simulink library "VIS_LIB"  (Simulink 8.6)
settings: Solver=ode45  StartTime=0.0  StopTime=10.0  RelTol=1e-3
undefined symbols (not defined in the file): AC, SIXOSEM_F_WD_AC_MASTER
libraries: cdsFilt x376, cdsEpicsOut x253, cdsEpicsIn x179, cdsTP x123, VIS_LIB x95, cdsMuxMatrix x91, cdsEpicsStringIn x75, cdsFiltCtrl x72, cdsFunctionCall x70, cdsRms x59, KAGRA_UTIL x25, STATE_BIO_MASTER x5
(part 5 of 38)

== system VIS_LIB/OLDAMP ==
  note: 1 (one) if GOOD
      | 0 (zero) if BAD
  PITCH_In : Inport
  YAW_In : Inport  Port=2
  Ground{1..2,4..5} (4 alike) : Ground
  Operator4 : RelationalOperator  Operator===  OutDataTypeStr=boolean
  Operator5 : RelationalOperator  Operator===  OutDataTypeStr=boolean
  P : cdsFiltCtrl/IIR FM with control  Tag=cdsFiltCtrl  Description=|
      | cdsFiltCntrl is the standard IIR filter module (exactly the same as cdsFilt) but with added control data output 'Ctrl'. Filter module digital signal output appears on the first output, which is called 'Val'. 'Ctrl' output has a bit pattern encoding the state of filter's on/off switches (FM1 through FM10). The bit values are:
      |                                                                                                                                                                                                                                                                                                                                       
      | module 	hex	dec                                                                                                                                                                                                                                                                                                                       
      | -----------------------                                                                                                                                                                                                                                                                                                               
      | FM1	0x20                    32                                                                                                                                                                                                                                                                                                        
      | FM2	0x80                     128                                                                                                                                                                                                                                                                                                      
      | FM3	0x200                   512                                                                                                                                                                                                                                                                                                       
      | FM4	0x800                   2048                                                                                                                                                                                                                                                                                                      
      | FM5	0x2000                 8192                                                                                                                                                                                                                                                                                                       
      | FM6	0x8000                 32768                                                                                                                                                                                                                                                                                                      
      | FM7	0x20000                131072                                                                                                                                                                                                                                                                                                     
      | FM8	0x80000                 524288                                                                                                                                                                                                                                                                                                    
      | FM9	0x200000               2097152                                                                                                                                                                                                                                                                                                    
      | FM10	0x800000               8388608                                                                                                                                                                                                                                                                                                   
      |                                                                                                                                                                                                                                                                                                                                       
      | This bit data can be used to drive some other switches or it can be output using a binary I/O module.
      settings: AttributesFormatString=%<Tag>
  P_STATE_GOOD : cdsEpicsIn/Subsystem  Tag=cdsEpicsIn  Description=|
      | Purpose:                                                                              
      | Create an EPICS input channel connection to the FE realtime controls.                 
      |                                                                                       
      | Operation:                                                                            
      | Outputs value from an EPICS ai record. Value is floating point with a precision of 3..
      |                                                                                       
      | Usage:                                                                                
      | Name the part with the desired EPICS channel name.
      settings: AttributesFormatString=%<Tag>
  P_STATE_NOW : cdsEpicsOut/Subsystem  Tag=cdsEpicsOutput  Description=|
      | Purpose:                                          
      | Output a FE signal to an EPICS channel.           
      |                                                   
      | Operation:                                        
      | Takes input value and passes it to EPICS record.  
      |                                                   
      | Usage:                                            
      | Name the part with the desired EPICS rrecord name.
      settings: AttributesFormatString=%<Tag>
  P_STATE_OK : cdsEpicsOut/Subsystem  Tag=cdsEpicsOutput  Description=|
      | Purpose:                                          
      | Output a FE signal to an EPICS channel.           
      |                                                   
      | Operation:                                        
      | Takes input value and passes it to EPICS record.  
      |                                                   
      | Usage:                                            
      | Name the part with the desired EPICS rrecord name.
      settings: AttributesFormatString=%<Tag>
  Product : Product  RndMeth=Zero
  STATE_OK : cdsEpicsOut/Subsystem  Tag=cdsEpicsOutput  Description=|
      | Purpose:                                          
      | Output a FE signal to an EPICS channel.           
      |                                                   
      | Operation:                                        
      | Takes input value and passes it to EPICS record.  
      |                                                   
      | Usage:                                            
      | Name the part with the desired EPICS rrecord name.
      settings: AttributesFormatString=%<Tag>
  Y : cdsFiltCtrl/IIR FM with control  Tag=cdsFiltCtrl  Description=|
      | cdsFiltCntrl is the standard IIR filter module (exactly the same as cdsFilt) but with added control data output 'Ctrl'. Filter module digital signal output appears on the first output, which is called 'Val'. 'Ctrl' output has a bit pattern encoding the state of filter's on/off switches (FM1 through FM10). The bit values are:
      |                                                                                                                                                                                                                                                                                                                                       
      | module 	hex	dec                                                                                                                                                                                                                                                                                                                       
      | -----------------------                                                                                                                                                                                                                                                                                                               
      | FM1	0x20                    32                                                                                                                                                                                                                                                                                                        
      | FM2	0x80                     128                                                                                                                                                                                                                                                                                                      
      | FM3	0x200                   512                                                                                                                                                                                                                                                                                                       
      | FM4	0x800                   2048                                                                                                                                                                                                                                                                                                      
      | FM5	0x2000                 8192                                                                                                                                                                                                                                                                                                       
      | FM6	0x8000                 32768                                                                                                                                                                                                                                                                                                      
      | FM7	0x20000                131072                                                                                                                                                                                                                                                                                                     
      | FM8	0x80000                 524288                                                                                                                                                                                                                                                                                                    
      | FM9	0x200000               2097152                                                                                                                                                                                                                                                                                                    
      | FM10	0x800000               8388608                                                                                                                                                                                                                                                                                                   
      |                                                                                                                                                                                                                                                                                                                                       
      | This bit data can be used to drive some other switches or it can be output using a binary I/O module.
      settings: AttributesFormatString=%<Tag>
  Y_STATE_GOOD : cdsEpicsIn/Subsystem  Tag=cdsEpicsIn  Description=|
      | Purpose:                                                                              
      | Create an EPICS input channel connection to the FE realtime controls.                 
      |                                                                                       
      | Operation:                                                                            
      | Outputs value from an EPICS ai record. Value is floating point with a precision of 3..
      |                                                                                       
      | Usage:                                                                                
      | Name the part with the desired EPICS channel name.
      settings: AttributesFormatString=%<Tag>
  Y_STATE_NOW : cdsEpicsOut/Subsystem  Tag=cdsEpicsOutput  Description=|
      | Purpose:                                          
      | Output a FE signal to an EPICS channel.           
      |                                                   
      | Operation:                                        
      | Takes input value and passes it to EPICS record.  
      |                                                   
      | Usage:                                            
      | Name the part with the desired EPICS rrecord name.
      settings: AttributesFormatString=%<Tag>
  Y_STATE_OK : cdsEpicsOut/Subsystem  Tag=cdsEpicsOutput  Description=|
      | Purpose:                                          
      | Output a FE signal to an EPICS channel.           
      |                                                   
      | Operation:                                        
      | Takes input value and passes it to EPICS record.  
      |                                                   
      | Usage:                                            
      | Name the part with the desired EPICS rrecord name.
      settings: AttributesFormatString=%<Tag>
  PITCH_Out : Outport
  YAW_Out : Outport  Port=2
  OLDAMP_STATE_Out : Outport  Port=3
  wires:
  Ground2/1 -> Y/3
  Ground1/1 -> P/3
  P/1 -> PITCH_Out/1
  Ground4/1 -> P/2
  PITCH_In/1 -> P/1
  P_STATE_GOOD/1 -> Operator4/1
  P/2 -> P_STATE_NOW/1
  Ground5/1 -> Y/2
  YAW_In/1 -> Y/1
  Y_STATE_GOOD/1 -> Operator5/1
  Y/2 -> Y_STATE_NOW/1
  Y/1 -> YAW_Out/1
  Operator4/1 -> P_STATE_OK/1
  Operator5/1 -> Y_STATE_OK/1
  Product/1 -> STATE_OK/1
  P_STATE_NOW/1 -> Operator4/2
  Y_STATE_NOW/1 -> Operator5/2
  STATE_OK/1 -> OLDAMP_STATE_Out/1
  P_STATE_OK/1 -> Product/1
  Y_STATE_OK/1 -> Product/2

== system VIS_LIB/OLDCCTRL ==
  note: 1 (one) if GOOD
      | 0 (zero) if BAD
  PITCH_In : Inport
  YAW_In : Inport  Port=2
  Ground{1..2,4..5} (4 alike) : Ground
  Operator4 : RelationalOperator  Operator===  OutDataTypeStr=boolean
  Operator5 : RelationalOperator  Operator===  OutDataTypeStr=boolean
  P : cdsFiltCtrl/IIR FM with control  Tag=cdsFiltCtrl  Description=|
      | cdsFiltCntrl is the standard IIR filter module (exactly the same as cdsFilt) but with added control data output 'Ctrl'. Filter module digital signal output appears on the first output, which is called 'Val'. 'Ctrl' output has a bit pattern encoding the state of filter's on/off switches (FM1 through FM10). The bit values are:
      |                                                                                                                                                                                                                                                                                                                                       
      | module 	hex	dec                                                                                                                                                                                                                                                                                                                       
      | -----------------------                                                                                                                                                                                                                                                                                                               
      | FM1	0x20                    32                                                                                                                                                                                                                                                                                                        
      | FM2	0x80                     128                                                                                                                                                                                                                                                                                                      
      | FM3	0x200                   512                                                                                                                                                                                                                                                                                                       
      | FM4	0x800                   2048                                                                                                                                                                                                                                                                                                      
      | FM5	0x2000                 8192                                                                                                                                                                                                                                                                                                       
      | FM6	0x8000                 32768                                                                                                                                                                                                                                                                                                      
      | FM7	0x20000                131072                                                                                                                                                                                                                                                                                                     
      | FM8	0x80000                 524288                                                                                                                                                                                                                                                                                                    
      | FM9	0x200000               2097152                                                                                                                                                                                                                                                                                                    
      | FM10	0x800000               8388608                                                                                                                                                                                                                                                                                                   
      |                                                                                                                                                                                                                                                                                                                                       
      | This bit data can be used to drive some other switches or it can be output using a binary I/O module.
      settings: AttributesFormatString=%<Tag>
  P_STATE_GOOD : cdsEpicsIn/Subsystem  Tag=cdsEpicsIn  Description=|
      | Purpose:                                                                              
      | Create an EPICS input channel connection to the FE realtime controls.                 
      |                                                                                       
      | Operation:                                                                            
      | Outputs value from an EPICS ai record. Value is floating point with a precision of 3..
      |                                                                                       
      | Usage:                                                                                
      | Name the part with the desired EPICS channel name.
      settings: AttributesFormatString=%<Tag>
  P_STATE_NOW : cdsEpicsOut/Subsystem  Tag=cdsEpicsOutput  Description=|
      | Purpose:                                          
      | Output a FE signal to an EPICS channel.           
      |                                                   
      | Operation:                                        
      | Takes input value and passes it to EPICS record.  
      |                                                   
      | Usage:                                            
      | Name the part with the desired EPICS rrecord name.
      settings: AttributesFormatString=%<Tag>
  P_STATE_OK : cdsEpicsOut/Subsystem  Tag=cdsEpicsOutput  Description=|
      | Purpose:                                          
      | Output a FE signal to an EPICS channel.           
      |                                                   
      | Operation:                                        
      | Takes input value and passes it to EPICS record.  
      |                                                   
      | Usage:                                            
      | Name the part with the desired EPICS rrecord name.
      settings: AttributesFormatString=%<Tag>
  Product : Product  RndMeth=Zero
  STATE_OK : cdsEpicsOut/Subsystem  Tag=cdsEpicsOutput  Description=|
      | Purpose:                                          
      | Output a FE signal to an EPICS channel.           
      |                                                   
      | Operation:                                        
      | Takes input value and passes it to EPICS record.  
      |                                                   
      | Usage:                                            
      | Name the part with the desired EPICS rrecord name.
      settings: AttributesFormatString=%<Tag>
  Y : cdsFiltCtrl/IIR FM with control  Tag=cdsFiltCtrl  Description=|
      | cdsFiltCntrl is the standard IIR filter module (exactly the same as cdsFilt) but with added control data output 'Ctrl'. Filter module digital signal output appears on the first output, which is called 'Val'. 'Ctrl' output has a bit pattern encoding the state of filter's on/off switches (FM1 through FM10). The bit values are:
      |                                                                                                                                                                                                                                                                                                                                       
      | module 	hex	dec                                                                                                                                                                                                                                                                                                                       
      | -----------------------                                                                                                                                                                                                                                                                                                               
      | FM1	0x20                    32                                                                                                                                                                                                                                                                                                        
      | FM2	0x80                     128                                                                                                                                                                                                                                                                                                      
      | FM3	0x200                   512                                                                                                                                                                                                                                                                                                       
      | FM4	0x800                   2048                                                                                                                                                                                                                                                                                                      
      | FM5	0x2000                 8192                                                                                                                                                                                                                                                                                                       
      | FM6	0x8000                 32768                                                                                                                                                                                                                                                                                                      
      | FM7	0x20000                131072                                                                                                                                                                                                                                                                                                     
      | FM8	0x80000                 524288                                                                                                                                                                                                                                                                                                    
      | FM9	0x200000               2097152                                                                                                                                                                                                                                                                                                    
      | FM10	0x800000               8388608                                                                                                                                                                                                                                                                                                   
      |                                                                                                                                                                                                                                                                                                                                       
      | This bit data can be used to drive some other switches or it can be output using a binary I/O module.
      settings: AttributesFormatString=%<Tag>
  Y_STATE_GOOD : cdsEpicsIn/Subsystem  Tag=cdsEpicsIn  Description=|
      | Purpose:                                                                              
      | Create an EPICS input channel connection to the FE realtime controls.                 
      |                                                                                       
      | Operation:                                                                            
      | Outputs value from an EPICS ai record. Value is floating point with a precision of 3..
      |                                                                                       
      | Usage:                                                                                
      | Name the part with the desired EPICS channel name.
      settings: AttributesFormatString=%<Tag>
  Y_STATE_NOW : cdsEpicsOut/Subsystem  Tag=cdsEpicsOutput  Description=|
      | Purpose:                                          
      | Output a FE signal to an EPICS channel.           
      |                                                   
      | Operation:                                        
      | Takes input value and passes it to EPICS record.  
      |                                                   
      | Usage:                                            
      | Name the part with the desired EPICS rrecord name.
      settings: AttributesFormatString=%<Tag>
  Y_STATE_OK : cdsEpicsOut/Subsystem  Tag=cdsEpicsOutput  Description=|
      | Purpose:                                          
      | Output a FE signal to an EPICS channel.           
      |                                                   
      | Operation:                                        
      | Takes input value and passes it to EPICS record.  
      |                                                   
      | Usage:                                            
      | Name the part with the desired EPICS rrecord name.
      settings: AttributesFormatString=%<Tag>
  PITCH_Out : Outport
  YAW_Out : Outport  Port=2
  OLDCCTRL_STATE_Out : Outport  Port=3
  wires:
  Ground2/1 -> Y/3
  Ground1/1 -> P/3
  P/1 -> PITCH_Out/1
  Ground4/1 -> P/2
  PITCH_In/1 -> P/1
  P_STATE_GOOD/1 -> Operator4/1
  P/2 -> P_STATE_NOW/1
  Ground5/1 -> Y/2
  YAW_In/1 -> Y/1
  Y_STATE_GOOD/1 -> Operator5/1
  Y/2 -> Y_STATE_NOW/1
  Y/1 -> YAW_Out/1
  Operator4/1 -> P_STATE_OK/1
  Operator5/1 -> Y_STATE_OK/1
  Product/1 -> STATE_OK/1
  P_STATE_NOW/1 -> Operator4/2
  Y_STATE_NOW/1 -> Operator5/2
  STATE_OK/1 -> OLDCCTRL_STATE_Out/1
  P_STATE_OK/1 -> Product/1
  Y_STATE_OK/1 -> Product/2

== system VIS_LIB/OPLEV_BLRMS_DOF ==
  In1 : Inport
  100M_300M : cdsEpicsOut/Subsystem  Tag=cdsEpicsOutput  Description=|
      | Purpose:                                          
      | Output a FE signal to an EPICS channel.           
      |                                                   
      | Operation:                                        
      | Takes input value and passes it to EPICS record.  
      |                                                   
      | Usage:                                            
      | Name the part with the desired EPICS rrecord name.
      settings: AttributesFormatString=%<Tag>
  10_30 : cdsEpicsOut/Subsystem  Tag=cdsEpicsOutput  Description=|
      | Purpose:                                          
      | Output a FE signal to an EPICS channel.           
      |                                                   
      | Operation:                                        
      | Takes input value and passes it to EPICS record.  
      |                                                   
      | Usage:                                            
      | Name the part with the desired EPICS rrecord name.
      settings: AttributesFormatString=%<Tag>
  1_3 : cdsEpicsOut/Subsystem  Tag=cdsEpicsOutput  Description=|
      | Purpose:                                          
      | Output a FE signal to an EPICS channel.           
      |                                                   
      | Operation:                                        
      | Takes input value and passes it to EPICS record.  
      |                                                   
      | Usage:                                            
      | Name the part with the desired EPICS rrecord name.
      settings: AttributesFormatString=%<Tag>
  300M_1 : cdsEpicsOut/Subsystem  Tag=cdsEpicsOutput  Description=|
      | Purpose:                                          
      | Output a FE signal to an EPICS channel.           
      |                                                   
      | Operation:                                        
      | Takes input value and passes it to EPICS record.  
      |                                                   
      | Usage:                                            
      | Name the part with the desired EPICS rrecord name.
      settings: AttributesFormatString=%<Tag>
  30M : cdsEpicsOut/Subsystem  Tag=cdsEpicsOutput  Description=|
      | Purpose:                                          
      | Output a FE signal to an EPICS channel.           
      |                                                   
      | Operation:                                        
      | Takes input value and passes it to EPICS record.  
      |                                                   
      | Usage:                                            
      | Name the part with the desired EPICS rrecord name.
      settings: AttributesFormatString=%<Tag>
  30M_100M : cdsEpicsOut/Subsystem  Tag=cdsEpicsOutput  Description=|
      | Purpose:                                          
      | Output a FE signal to an EPICS channel.           
      |                                                   
      | Operation:                                        
      | Takes input value and passes it to EPICS record.  
      |                                                   
      | Usage:                                            
      | Name the part with the desired EPICS rrecord name.
      settings: AttributesFormatString=%<Tag>
  30_100 : cdsEpicsOut/Subsystem  Tag=cdsEpicsOutput  Description=|
      | Purpose:                                          
      | Output a FE signal to an EPICS channel.           
      |                                                   
      | Operation:                                        
      | Takes input value and passes it to EPICS record.  
      |                                                   
      | Usage:                                            
      | Name the part with the desired EPICS rrecord name.
      settings: AttributesFormatString=%<Tag>
  3_10 : cdsEpicsOut/Subsystem  Tag=cdsEpicsOutput  Description=|
      | Purpose:                                          
      | Output a FE signal to an EPICS channel.           
      |                                                   
      | Operation:                                        
      | Takes input value and passes it to EPICS record.  
      |                                                   
      | Usage:                                            
      | Name the part with the desired EPICS rrecord name.
      settings: AttributesFormatString=%<Tag>
  BLRMS : cdsFunctionCall/Subsystem  Tag=cdsFunctionCall  Description=inline BLRMS /opt/rtcds/userapps/release/cds/common/src/BLRMSFILTER.c
      settings: AttributesFormatString=%<Tag>\n%<Description>
  Constant2 : Constant  Value=2
  Demux : Demux  Outputs=8
  Mux : Mux  Inputs=2
  Terminator{1..8} (8 alike) : Terminator
  wires:
  BLRMS/1 -> Demux/1
  Mux/1 -> BLRMS/1
  In1/1 -> Mux/1
  Demux/1 -> 30M/1
  Demux/2 -> 30M_100M/1
  Demux/3 -> 100M_300M/1
  Demux/4 -> 300M_1/1
  Demux/5 -> 1_3/1
  Demux/6 -> 3_10/1
  Demux/7 -> 10_30/1
  Demux/8 -> 30_100/1
  30M/1 -> Terminator8/1
  30M_100M/1 -> Terminator1/1
  100M_300M/1 -> Terminator2/1
  300M_1/1 -> Terminator3/1
  1_3/1 -> Terminator4/1
  3_10/1 -> Terminator5/1
  10_30/1 -> Terminator6/1
  30_100/1 -> Terminator7/1
  Constant2/1 -> Mux/2

== system VIS_LIB/PAY_OLSERVO ==
  OL_MNP_In : Inport
  OL_MNY_In : Inport  Port=2
  OL_TML_In : Inport  Port=3
  OL_TMP_In : Inport  Port=4
  OL_TMY_In : Inport  Port=5
  ADD : Subsystem
  DAMP : Subsystem
  Demux1 : Demux  Outputs=24
  Demux2 : Demux  Outputs=10
  Mux1 : Mux  Inputs=24
  Mux2 : Mux  Inputs=5
  OL2PK : cdsMuxMatrix/Subsystem  Tag=cdsMuxMatrix  Description=Any size matrix. Inputs and outputs must be connected using Mux and Demux parts.
      settings: AttributesFormatString=%<Tag>
  PK2EUL : cdsMuxMatrix/Subsystem  Tag=cdsMuxMatrix  Description=Any size matrix. Inputs and outputs must be connected using Mux and Demux parts.
      settings: AttributesFormatString=%<Tag>
  PKOUT : Subsystem
  TEST : Subsystem
  BFY_Out : Outport
  MNL_Out : Outport  Port=2
  MNP_Out : Outport  Port=3
  MNY_Out : Outport  Port=4
  IML_Out : Outport  Port=5
  IMP_Out : Outport  Port=6
  IMY_Out : Outport  Port=7
  TML_Out : Outport  Port=8
  TMP_Out : Outport  Port=9
  TMY_Out : Outport  Port=10
  wires:
  OL_TMP_In/1 -> Mux2/4
  OL_TMY_In/1 -> Mux2/5
  OL_MNP_In/1 -> Mux2/1
  OL_MNY_In/1 -> Mux2/2
  OL_TML_In/1 -> Mux2/3
  Mux2/1 -> OL2PK/1
  OL2PK/1 -> Demux1/1
  Demux1/3 -> DAMP/3(P03_In)
  Demux1/6 -> DAMP/6(P06_In)
  Demux1/4 -> DAMP/4(P04_In)
  Demux1/1 -> DAMP/1(P01_In)
  Demux1/2 -> DAMP/2(P02_In)
  Demux1/7 -> DAMP/7(P07_In)
  Demux1/8 -> DAMP/8(P08_In)
  Demux1/9 -> DAMP/9(P09_In)
  Demux1/10 -> DAMP/10(P10_In)
  Demux1/11 -> DAMP/11(P11_In)
  Demux1/12 -> DAMP/12(P12_In1)
  Demux1/5 -> DAMP/5(P05_In)
  TEST/12(P12_Out) -> ADD/12(TEST_P12_In)
  TEST/6(P06_Out) -> ADD/6(TEST_P06_In)
  TEST/7(P07_Out) -> ADD/7(TEST_P07_In)
  TEST/8(P08_Out) -> ADD/8(TEST_P08_In)
  TEST/9(P09_Out) -> ADD/9(TEST_P09_In)
  TEST/10(P10_Out) -> ADD/10(TEST_P10_In)
  TEST/11(P11_Out) -> ADD/11(TEST_P11_In)
  TEST/1(P01_Out) -> ADD/1(TEST_P01_In)
  TEST/2(P02_Out) -> ADD/2(TEST_P02_In)
  TEST/3(P03_Out) -> ADD/3(TEST_P03_In)
  TEST/4(P04_Out) -> ADD/4(TEST_P04_In)
  TEST/5(P05_Out) -> ADD/5(TEST_P05_In)
  DAMP/11(P11_Out) -> ADD/35(DAMP_P11_In)
  DAMP/4(P04_Out) -> ADD/28(DAMP_P04_In)
  DAMP/5(P05_Out) -> ADD/29(DAMP_P05_In)
  DAMP/6(P06_Out) -> ADD/30(DAMP_P06_In)
  DAMP/12(P12_Out) -> ADD/36(DAMP_P12_In)
  DAMP/8(P08_Out) -> ADD/32(DAMP_P08_In)
  DAMP/10(P10_Out) -> ADD/34(DAMP_P10_In)
  DAMP/7(P07_Out) -> ADD/31(DAMP_P07_In)
  DAMP/9(P09_Out) -> ADD/33(DAMP_P09_In)
  DAMP/1(P01_Out) -> ADD/25(DAMP_P01_In)
  DAMP/2(P02_Out) -> ADD/26(DAMP_P02_In)
  DAMP/3(P03_Out) -> ADD/27(DAMP_P03_In)
  Mux1/1 -> PK2EUL/1
  PK2EUL/1 -> Demux2/1
  Demux2/3 -> MNP_Out/1
  Demux2/1 -> BFY_Out/1
  Demux2/2 -> MNL_Out/1
  Demux2/10 -> TMY_Out/1
  Demux2/8 -> TML_Out/1
  Demux2/4 -> MNY_Out/1
  Demux2/9 -> TMP_Out/1
  Demux2/7 -> IMY_Out/1
  Demux2/5 -> IML_Out/1
  Demux2/6 -> IMP_Out/1
  Demux1/13 -> DAMP/13(P13_In)
  Demux1/14 -> DAMP/14(P14_In)
  Demux1/15 -> DAMP/15(P15_In)
  Demux1/16 -> DAMP/16(P16_In)
  Demux1/17 -> DAMP/17(P17_In)
  Demux1/18 -> DAMP/18(P18_In)
  Demux1/19 -> DAMP/19(P19_In)
  Demux1/20 -> DAMP/20(P20_In)
  Demux1/21 -> DAMP/21(P21_In)
  Demux1/22 -> DAMP/22(P22_In)
  Demux1/23 -> DAMP/23(P23_In)
  Demux1/24 -> DAMP/24(P24_In)
  TEST/13(P13_Out) -> ADD/13(TEST_P13_In)
  TEST/14(P14_Out) -> ADD/14(TEST_P14_In)
  TEST/15(P15_Out) -> ADD/15(TEST_P15_In)
  TEST/16(P16_Out) -> ADD/16(TEST_P16_In)
  TEST/17(P17_Out) -> ADD/17(TEST_P17_In)
  TEST/18(P18_Out) -> ADD/18(TEST_P18_In)
  TEST/19(P19_Out) -> ADD/19(TEST_P19_In)
  TEST/20(P20_Out) -> ADD/20(TEST_P20_In)
  TEST/21(P21_Out) -> ADD/21(TEST_P21_In)
  TEST/22(P22_Out) -> ADD/22(TEST_P22_In)
  TEST/23(P23_Out) -> ADD/23(TEST_P23_In)
  TEST/24(P24_Out) -> ADD/24(TEST_P24_In)
  DAMP/13(P13_Out) -> ADD/37(DAMP_P13_In)
  DAMP/14(P14_Out) -> ADD/38(DAMP_P14_In)
  DAMP/15(P15_Out) -> ADD/39(DAMP_P15_In)
  DAMP/16(P16_Out) -> ADD/40(DAMP_P16_In)
  DAMP/17(P17_Out) -> ADD/41(DAMP_P17_In)
  DAMP/18(P18_Out) -> ADD/42(DAMP_P18_In)
  DAMP/19(P19_Out) -> ADD/43(DAMP_P19_In)
  DAMP/20(P20_Out) -> ADD/44(DAMP_P20_In)
  DAMP/21(P21_Out) -> ADD/45(DAMP_P21_In)
  DAMP/22(P22_Out) -> ADD/46(DAMP_P22_In)
  DAMP/23(P23_Out) -> ADD/47(DAMP_P23_In)
  DAMP/24(P24_Out) -> ADD/48(DAMP_P24_In)
  ADD/16(P16_Out) -> PKOUT/16(P16_In), Mux1/16
  ADD/14(P14_Out) -> PKOUT/14(P14_In), Mux1/14
  ADD/19(P19_Out) -> PKOUT/19(P19_In), Mux1/19
  ADD/20(P20_Out) -> PKOUT/20(P20_In), Mux1/20
  ADD/24(P24_Out) -> PKOUT/24(P24_In), Mux1/24
  ADD/22(P22_Out) -> PKOUT/22(P22_In), Mux1/22
  ADD/23(P23_Out) -> PKOUT/23(P23_In), Mux1/23
  ADD/13(P13_Out) -> PKOUT/13(P13_In), Mux1/13
  ADD/15(P15_Out) -> PKOUT/15(P15_In), Mux1/15
  ADD/2(P02_Out) -> PKOUT/2(P02_In), Mux1/2
  ADD/3(P03_Out) -> PKOUT/3(P03_In), Mux1/3
  ADD/4(P04_Out) -> PKOUT/4(P04_In), Mux1/4
  ADD/5(P05_Out) -> PKOUT/5(P05_In), Mux1/5
  ADD/6(P06_Out) -> PKOUT/6(P06_In), Mux1/6
  ADD/7(P07_Out) -> PKOUT/7(P07_In), Mux1/7
  ADD/8(P08_Out) -> PKOUT/8(P08_In), Mux1/8
  ADD/9(P09_Out) -> PKOUT/9(P09_In), Mux1/9
  ADD/10(P10_Out) -> PKOUT/10(P10_In), Mux1/10
  ADD/11(P11_Out) -> PKOUT/11(P11_In), Mux1/11
  ADD/12(P12_Out) -> PKOUT/12(P12_In), Mux1/12
  ADD/17(P17_Out) -> PKOUT/17(P17_In), Mux1/17
  ADD/18(P18_Out) -> PKOUT/18(P18_In), Mux1/18
  ADD/21(P21_Out) -> PKOUT/21(P21_In), Mux1/21
  ADD/1(P01_Out) -> PKOUT/1(P01_In), Mux1/1
